simulink library "Electrical_charger"  (R2016a)
settings: Solver=ode45  StartTime=0.0  StopTime=10.0  RelTol=1e-3
undefined symbols (not defined in the file): AWR_InvStError, Charger, Charger_resistance, CONST_POWER_ERR_MODE, drvEmot_AWR_InvStError, SIGVAL_STATUS_ERROR
libraries: simulink x5
settings Model: Creator=krishs1  LastModifiedBy=krishs1
settings DataIOCC: LimitDataPoints=on
settings DebuggingCC: AllowSymbolicDim=off

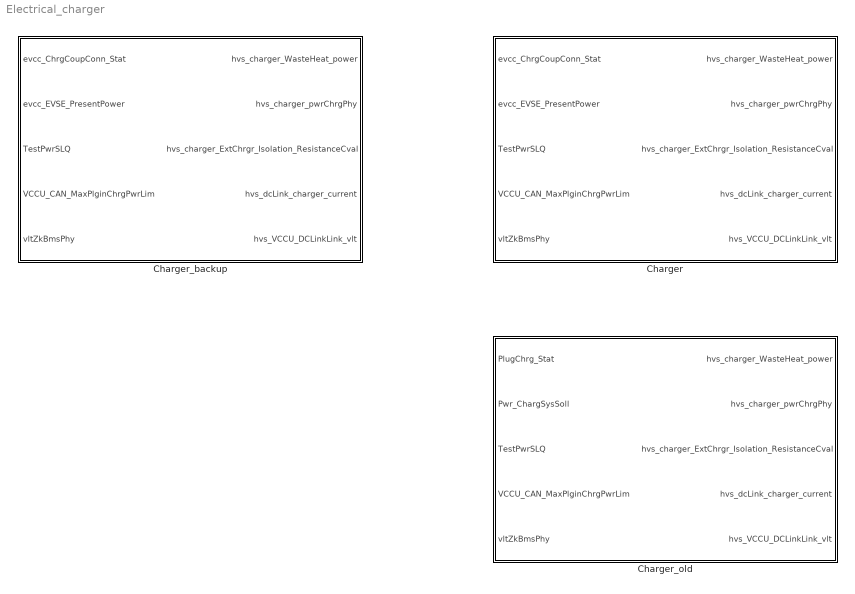
== system Electrical_charger ==
  Charger : Subsystem
  Charger_backup : Subsystem
  Charger_old : Subsystem

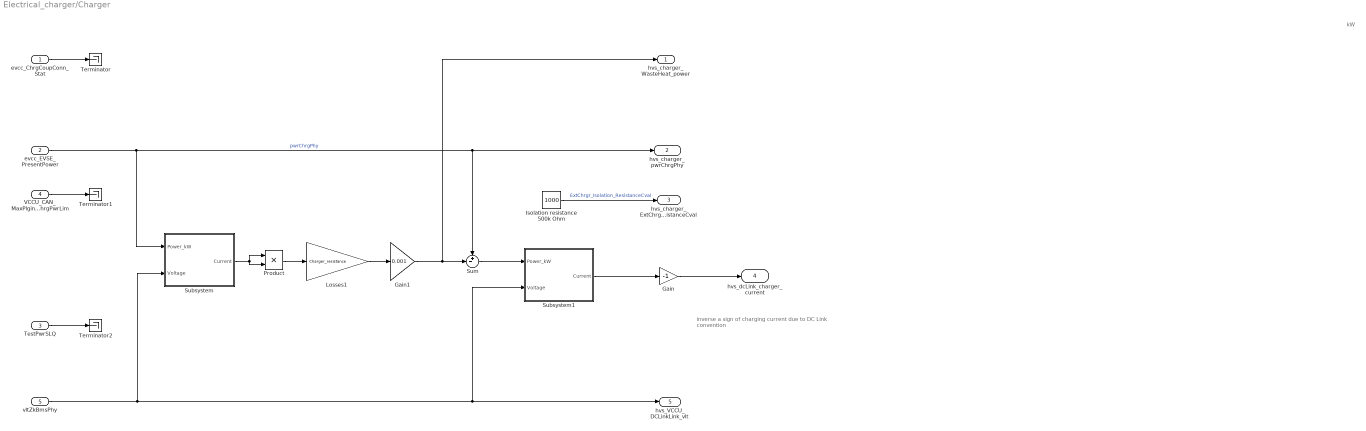
== system Electrical_charger/Charger ==
  note: kW
  note: inverse a sign of charging current due to DC Link
      | convention
  evcc_ChrgCoupConn_Stat : Inport
  evcc_EVSE_PresentPower : Inport  Port=2
  TestPwrSLQ : Inport  Port=3
  VCCU_CAN_MaxPlginChrgPwrLim : Inport  Port=4
  vltZkBmsPhy : Inport  Port=5
  Gain : Gain  Gain=-1
  Gain1 : Gain  Gain=0.001
  Isolation resistance 500k Ohm : Constant  Value=1000
  Losses1 : Gain  Gain=Charger_resistance
  Product : Product
  Subsystem : Subsystem
  Subsystem1 : Subsystem
  Sum : Sum  Inputs=+-|
  Terminator : Terminator
  Terminator1 : Terminator
  Terminator2 : Terminator
  hvs_charger_WasteHeat_power : Outport
  hvs_charger_pwrChrgPhy : Outport  Port=2
  hvs_charger_ExtChrgr_Isolation_ResistanceCval : Outport  Port=3
  hvs_dcLink_charger_current : Outport  Port=4
  hvs_VCCU_DCLinkLink_vlt : Outport  Port=5
  wires:
  evcc_EVSE_PresentPower/1 -> Sum/1, hvs_charger_pwrChrgPhy/1, Subsystem/1(Power_kW)  "pwrChrgPhy"
  Isolation resistance 500k Ohm/1 -> hvs_charger_ExtChrgr_Isolation_ResistanceCval/1  "ExtChrgr_Isolation_ResistanceCval"
  vltZkBmsPhy/1 -> Subsystem1/2(Voltage), hvs_VCCU_DCLinkLink_vlt/1, Subsystem/2(Voltage)
  evcc_ChrgCoupConn_Stat/1 -> Terminator/1
  VCCU_CAN_MaxPlginChrgPwrLim/1 -> Terminator1/1
  TestPwrSLQ/1 -> Terminator2/1
  Gain/1 -> hvs_dcLink_charger_current/1
  Subsystem1/1(Current) -> Gain/1
  Product/1 -> Losses1/1
  Losses1/1 -> Gain1/1
  Gain1/1 -> hvs_charger_WasteHeat_power/1, Sum/2
  Sum/1 -> Subsystem1/1(Power_kW)
  Subsystem/1(Current) -> Product/1, Product/2

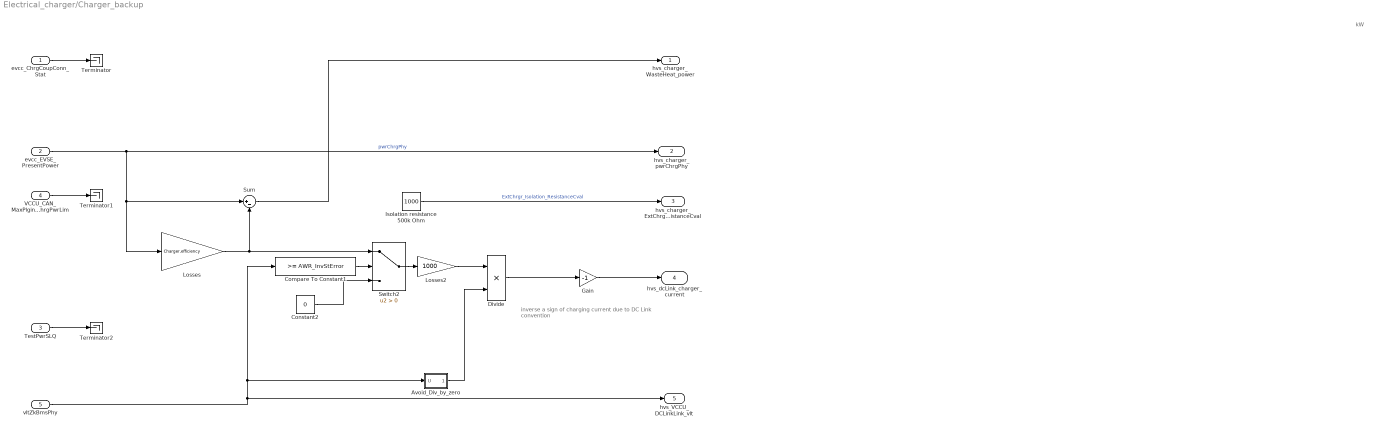
== system Electrical_charger/Charger_backup ==
  note: inverse a sign of charging current due to DC Link
      | convention
  note: kW
  evcc_ChrgCoupConn_Stat : Inport
  evcc_EVSE_PresentPower : Inport  Port=2
  TestPwrSLQ : Inport  Port=3
  VCCU_CAN_MaxPlginChrgPwrLim : Inport  Port=4
  vltZkBmsPhy : Inport  Port=5
  Avoid_Div_by_zero : Subsystem
  Compare To Constant1 : simulink/Logic and Bit Operations/Compare To Constant  relop=>=  const=AWR_InvStError  OutDataTypeStr=boolean
  Constant2 : Constant  Value=0
  Divide : Product  Inputs=**
  Gain : Gain  Gain=-1
  Isolation resistance 500k Ohm : Constant  Value=1000
  Losses : Gain  Gain=Charger.efficiency
  Losses2 : Gain  Gain=1000
  Sum : Sum  Inputs=|+-
  Switch2 : Switch  Criteria=u2 > Threshold
  Terminator : Terminator
  Terminator1 : Terminator
  Terminator2 : Terminator
  hvs_charger_WasteHeat_power : Outport
  hvs_charger_pwrChrgPhy : Outport  Port=2
  hvs_charger_ExtChrgr_Isolation_ResistanceCval : Outport  Port=3
  hvs_dcLink_charger_current : Outport  Port=4
  hvs_VCCU_DCLinkLink_vlt : Outport  Port=5
  wires:
  Divide/1 -> Gain/1
  Avoid_Div_by_zero/1(1/U) -> Divide/2
  evcc_EVSE_PresentPower/1 -> Losses/1, Sum/1, hvs_charger_pwrChrgPhy/1  "pwrChrgPhy"
  Isolation resistance 500k Ohm/1 -> hvs_charger_ExtChrgr_Isolation_ResistanceCval/1  "ExtChrgr_Isolation_ResistanceCval"
  Losses2/1 -> Divide/1
  Losses/1 -> Sum/2, Switch2/1
  Sum/1 -> hvs_charger_WasteHeat_power/1
  Compare To Constant1/1 -> Switch2/2
  Constant2/1 -> Switch2/3
  vltZkBmsPhy/1 -> hvs_VCCU_DCLinkLink_vlt/1, Compare To Constant1/1, Avoid_Div_by_zero/1(U)
  Switch2/1 -> Losses2/1
  evcc_ChrgCoupConn_Stat/1 -> Terminator/1
  VCCU_CAN_MaxPlginChrgPwrLim/1 -> Terminator1/1
  TestPwrSLQ/1 -> Terminator2/1
  Gain/1 -> hvs_dcLink_charger_current/1

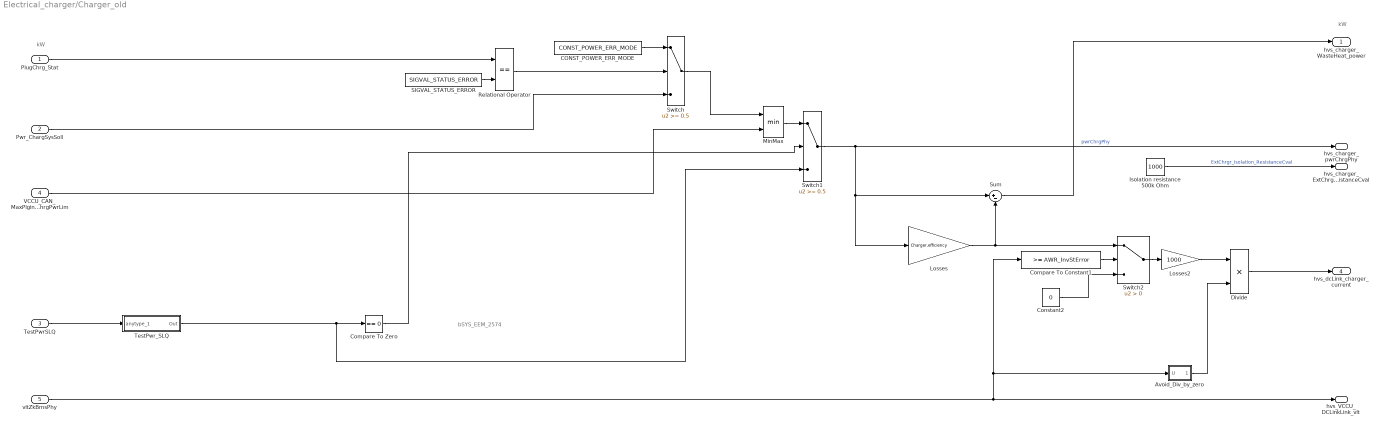
== system Electrical_charger/Charger_old ==
  note: bSYS_EEM_2574
  note: kW
  note: kW
  PlugChrg_Stat : Inport
  Pwr_ChargSysSoll : Inport  Port=2
  TestPwrSLQ : Inport  Port=3
  VCCU_CAN_MaxPlginChrgPwrLim : Inport  Port=4
  vltZkBmsPhy : Inport  Port=5
  Avoid_Div_by_zero : Subsystem
  CONST_POWER_ERR_MODE : Constant  Value=CONST_POWER_ERR_MODE
  Compare To Constant1 : simulink/Logic and Bit Operations/Compare To Constant  relop=>=  const=AWR_InvStError  OutDataTypeStr=boolean
  Compare To Zero : simulink/Logic and Bit Operations/Compare To Zero  relop===  OutDataTypeStr=boolean
  Constant2 : Constant  Value=0
  Divide : Product  Inputs=**
  Isolation resistance 500k Ohm : Constant  Value=1000
  Losses : Gain  Gain=Charger.efficiency
  Losses2 : Gain  Gain=1000
  MinMax : MinMax  Inputs=2
  Relational Operator : RelationalOperator  Operator===  OutDataTypeStr=boolean
  SIGVAL_STATUS_ERROR : Constant  Value=SIGVAL_STATUS_ERROR
  Sum : Sum  Inputs=|+-
  Switch : Switch  Threshold=0.5
  Switch1 : Switch  Threshold=0.5
  Switch2 : Switch  Criteria=u2 > Threshold
  TestPwr_SLQ : Subsystem  Tag=Manip_Signal  mask(TOI_ManipSignal){Attribute_String=, DataType_String=double(0)}
      mask prompts: Attribute_String "Attribute String"; DataType_String "DataType String"
      mask help: Manipulates a signal (breaks a loop). This block can be detected by PROVEtech:TA to display the four values (in, out, control, active) and all other data belonging to the signal (e.g. unit, description, min/max values...).
      mask init:
      | if isempty(Attribute_String)
      |   set_param([gcb '/Active'], 'Value', 'boolean(0)');
      |   strColor='black';
      |   strDesc='';
      | else
      |   [strDesc iPos]=strtokex(Attribute_String, 0);
      |   [strUnit iPos]=strtokex(Attribute_String, iPos);
      |   [strMin iPos]=strtokex(Attribute_String, iPos);
      |   [strMax iPos]=strtokex(Attribute_String, iPos);
      |   [strDef iPos]=strtokex(Attribute_String, iPos);
      |   [strAct iPos]=strtokex(Attribute_String, iPos);
      |   strColor='gray';
      |   active=evalin('base', strAct);
      |   strAct=mat2str(active);
      |   set_param([gcb '/Active'], 'Value', ['boolean(' strAct ')']);
      |   if any(active(:))
      | 	  strColor='red';
      |   else
      | 	  strColor='black';
      |   end;
      |   strDesc=sprintf('%s|%s|%s|%s|%s|%s%s', strDesc, strUnit, mat2str(evalin('base', strMin)), mat2str(evalin('base', strMax)), mat2str(evalin('base', strDef)), strAct, Attribute_String(iPos:length(Attribute_String)));
      | end
      | set_param([gcb '/Control'], 'Value', DataType_String);
      | set_param([gcb '/Control'], 'Description', strDesc);
      settings: OpenFcn=TOI_Block
      mask Display:
      | color(strColor);
      | disp(['Manip ' DataType_String]);
  hvs_charger_WasteHeat_power : Outport
  hvs_charger_pwrChrgPhy : Outport  Port=2
  hvs_charger_ExtChrgr_Isolation_ResistanceCval : Outport  Port=3
  hvs_dcLink_charger_current : Outport  Port=4
  hvs_VCCU_DCLinkLink_vlt : Outport  Port=5
  wires:
  Switch2/1 -> Losses2/1
  vltZkBmsPhy/1 -> hvs_VCCU_DCLinkLink_vlt/1, Avoid_Div_by_zero/1(U), Compare To Constant1/1
  Constant2/1 -> Switch2/3
  Compare To Constant1/1 -> Switch2/2
  Sum/1 -> hvs_charger_WasteHeat_power/1
  Losses/1 -> Switch2/1, Sum/2
  Losses2/1 -> Divide/1
  TestPwr_SLQ/1(Out) -> Compare To Zero/1, Switch1/3
  Isolation resistance 500k Ohm/1 -> hvs_charger_ExtChrgr_Isolation_ResistanceCval/1  "ExtChrgr_Isolation_ResistanceCval"
  Pwr_ChargSysSoll/1 -> Switch/3
  MinMax/1 -> Switch1/1
  Switch1/1 -> hvs_charger_pwrChrgPhy/1, Sum/1, Losses/1  "pwrChrgPhy"
  Compare To Zero/1 -> Switch1/2
  TestPwrSLQ/1 -> TestPwr_SLQ/1(anytype_1)
  VCCU_CAN_MaxPlginChrgPwrLim/1 -> MinMax/2
  Switch/1 -> MinMax/1
  CONST_POWER_ERR_MODE/1 -> Switch/1
  Relational Operator/1 -> Switch/2
  SIGVAL_STATUS_ERROR/1 -> Relational Operator/2
  PlugChrg_Stat/1 -> Relational Operator/1
  Avoid_Div_by_zero/1(1/U) -> Divide/2
  Divide/1 -> hvs_dcLink_charger_current/1

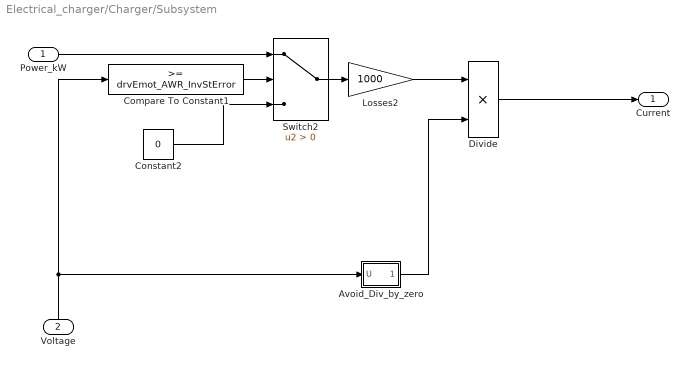
== system Electrical_charger/Charger/Subsystem ==
  Power_kW : Inport
  Voltage : Inport  Port=2
  Avoid_Div_by_zero : Subsystem
  Compare To Constant1 : simulink/Logic and Bit Operations/Compare To Constant  relop=>=  const=drvEmot_AWR_InvStError  OutDataTypeStr=boolean
  Constant2 : Constant  Value=0
  Divide : Product  Inputs=**
  Losses2 : Gain  Gain=1000
  Switch2 : Switch  Criteria=u2 > Threshold
  Current : Outport
  wires:
  Power_kW/1 -> Switch2/1
  Voltage/1 -> Compare To Constant1/1, Avoid_Div_by_zero/1(U)
  Avoid_Div_by_zero/1(1/U) -> Divide/2
  Losses2/1 -> Divide/1
  Compare To Constant1/1 -> Switch2/2
  Divide/1 -> Current/1
  Constant2/1 -> Switch2/3
  Switch2/1 -> Losses2/1

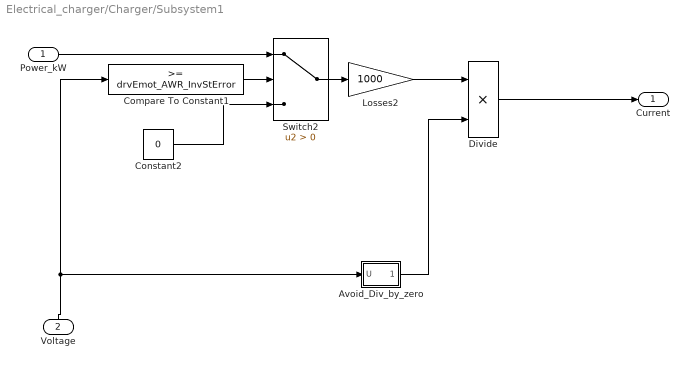
== system Electrical_charger/Charger/Subsystem1 ==
  Power_kW : Inport
  Voltage : Inport  Port=2
  Avoid_Div_by_zero : Subsystem
  Compare To Constant1 : simulink/Logic and Bit Operations/Compare To Constant  relop=>=  const=drvEmot_AWR_InvStError  OutDataTypeStr=boolean
  Constant2 : Constant  Value=0
  Divide : Product  Inputs=**
  Losses2 : Gain  Gain=1000
  Switch2 : Switch  Criteria=u2 > Threshold
  Current : Outport
  wires:
  Switch2/1 -> Losses2/1
  Constant2/1 -> Switch2/3
  Divide/1 -> Current/1
  Compare To Constant1/1 -> Switch2/2
  Losses2/1 -> Divide/1
  Avoid_Div_by_zero/1(1/U) -> Divide/2
  Voltage/1 -> Avoid_Div_by_zero/1(U), Compare To Constant1/1
  Power_kW/1 -> Switch2/1

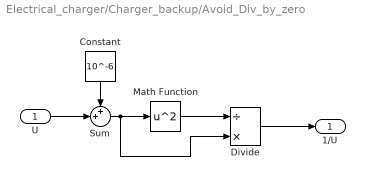
== system Electrical_charger/Charger_backup/Avoid_Div_by_zero ==
  U : Inport
  Constant : Constant  Value=10^-6
  Divide : Product  Inputs=/*
  Math Function : Math  Operator=square  SaturateOnIntegerOverflow=on
  Sum : Sum  Inputs=++|
  1/U : Outport
  wires:
  U/1 -> Sum/2
  Constant/1 -> Sum/1
  Sum/1 -> Math Function/1, Divide/2
  Math Function/1 -> Divide/1
  Divide/1 -> 1/U/1

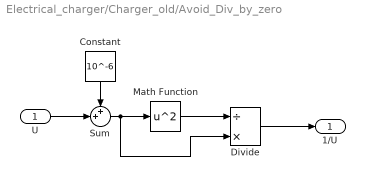
== system Electrical_charger/Charger_old/Avoid_Div_by_zero ==
  U : Inport
  Constant : Constant  Value=10^-6
  Divide : Product  Inputs=/*
  Math Function : Math  Operator=square  SaturateOnIntegerOverflow=on
  Sum : Sum  Inputs=++|
  1/U : Outport
  wires:
  Divide/1 -> 1/U/1
  Math Function/1 -> Divide/1
  Sum/1 -> Divide/2, Math Function/1
  Constant/1 -> Sum/1
  U/1 -> Sum/2

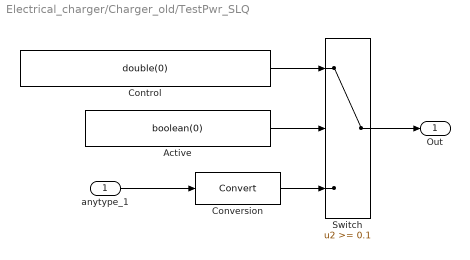
== system Electrical_charger/Charger_old/TestPwr_SLQ ==
  anytype_1 : Inport
  Active : Constant  Value=boolean(0)
  Control : Constant  Value=double(0)
  Conversion : DataTypeConversion  RndMeth=Zero
  Switch : Switch  Threshold=0.1  SaturateOnIntegerOverflow=on  InputSameDT=on
  Out : Outport  Description=||0|0|0
  wires:
  Switch/1 -> Out/1
  Conversion/1 -> Switch/3
  Active/1 -> Switch/2
  Control/1 -> Switch/1
  anytype_1/1 -> Conversion/1

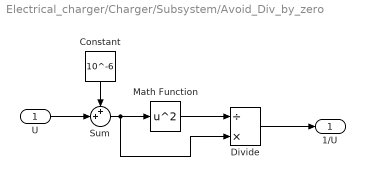
== system Electrical_charger/Charger/Subsystem/Avoid_Div_by_zero ==
  U : Inport
  Constant : Constant  Value=10^-6
  Divide : Product  Inputs=/*
  Math Function : Math  Operator=square  SaturateOnIntegerOverflow=on
  Sum : Sum  Inputs=++|
  1/U : Outport
  wires:
  U/1 -> Sum/2
  Constant/1 -> Sum/1
  Sum/1 -> Math Function/1, Divide/2
  Math Function/1 -> Divide/1
  Divide/1 -> 1/U/1

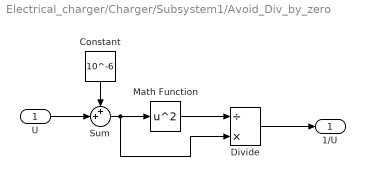
== system Electrical_charger/Charger/Subsystem1/Avoid_Div_by_zero ==
  U : Inport
  Constant : Constant  Value=10^-6
  Divide : Product  Inputs=/*
  Math Function : Math  Operator=square  SaturateOnIntegerOverflow=on
  Sum : Sum  Inputs=++|
  1/U : Outport
  wires:
  Divide/1 -> 1/U/1
  Math Function/1 -> Divide/1
  Sum/1 -> Divide/2, Math Function/1
  Constant/1 -> Sum/1
  U/1 -> Sum/2
